simulink model "task_4"  (R2023b)
settings: Solver=FixedStepDiscrete  StartTime=0.0  StopTime=(16+14)*16-1  RelTol=1e-3
libraries: dspsigops x2, commchan3 x1, dspstat3 x1, dspsrcs4 x1
settings Model: Creator=bhalaaj  LastModifiedBy=AMEY THAKUR

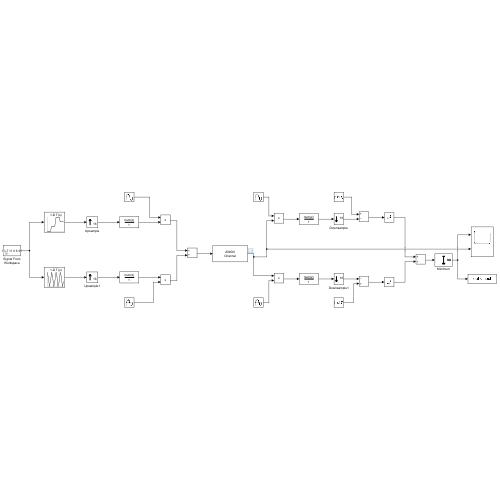
[thumbnail: Simulink's stored preview of the top-level diagram]
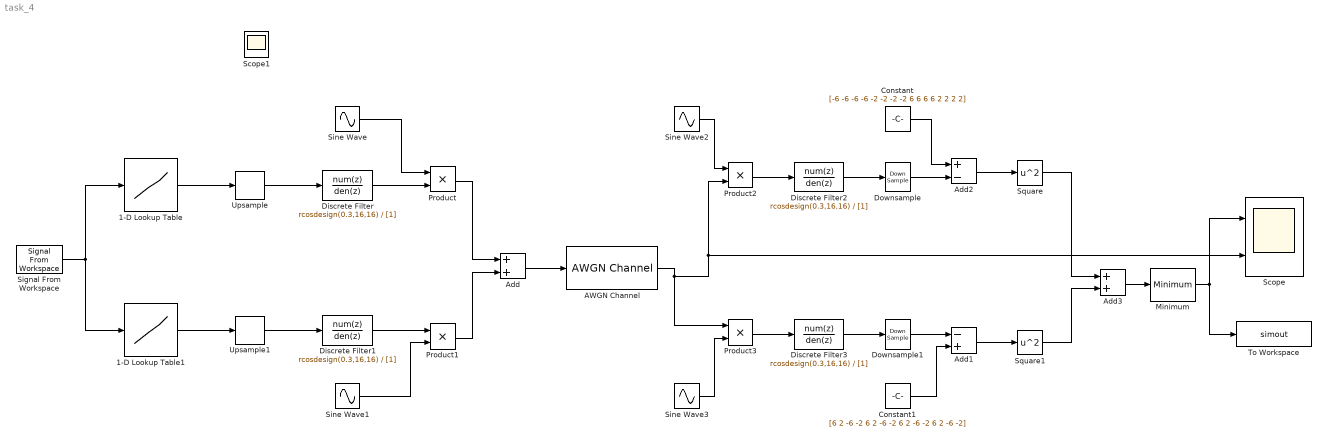
== system task_4 ==
  1-D Lookup Table : Lookup_n-D  NumberOfTableDimensions=1  BreakpointsForDimension1=[0:15]  Table=[-6 -6 -6 -6 -2 -2 -2 -2 6 6 6 6 2 2 2 2]  InternalRulePriority=Speed  RndMeth=Simplest
  1-D Lookup Table1 : Lookup_n-D  NumberOfTableDimensions=1  BreakpointsForDimension1=[0:15]  Table=[6 2 -6 -2 6 2 -6 -2 6 2 -6 -2 6 2 -6 -2]  InternalRulePriority=Speed  RndMeth=Simplest
  AWGN Channel : commchan3/AWGN Channel  LegacyMode=off  NoiseMethod="Signal to noise ratio  (Es/No)"  noiseMode="Signal to noise ratio  (SNR)"  EbNo=10  EsNo=40  SNR=10  BitsPerSymbol=1  SignalPower=1  SamplesPerSymbol=1  SymbolPeriod=1  VarianceSource=Parameter  Variance=1  RandomStream=mt19937ar with seed  Seed=110107589  SimulateUsing=Code generation
  Add : Sum
  Add1 : Sum  Inputs=-+
  Add2 : Sum  Inputs=+-
  Add3 : Sum
  Constant : Constant  Value=[-6 -6 -6 -6 -2 -2 -2 -2 6 6 6 6 2 2 2 2]
  Constant1 : Constant  Value=[6 2 -6 -2 6 2 -6 -2 6 2 -6 -2 6 2 -6 -2]
  Discrete Filter{,1..3} (4 alike) : DiscreteFilter  Numerator=rcosdesign(0.3,16,16)  Denominator=[1]
  Downsample : DownSample  N=16  RateOptions=Allow multirate processing
  Downsample1 : DownSample  N=16  RateOptions=Allow multirate processing
  Minimum : dspstat3/Minimum  operation=minimum  fcn=Index  indexBase=Zero  operateOver=Entire input  Dimension=1  InputProcessing=Columns as channels (frame based)  reset=None  roiEnable=off  roiType=Rectangles  roiPortion=Entire ROI  roiOutput=Individual statistics for each ROI  roiFlag=off  roundingMode=Floor  overflowMode=off
      settings: LibrarySourceBlock=dsphdlsupportstat/Minimum
  Product{,1..3} (4 alike) : Product
  Scope : Scope  NumInputPorts=2
  Signal From Workspace : dspsrcs4/Signal From Workspace  X=[15 13 10 3 7 11 0 6 9 3 1 2 4 5]  Ts=16  nsamps=1  OutputAfterFinalValue=Setting to zero  ignoreOrWarnInputAndFrameLengths=off  OutputFrames=off
  Sine Wave : Sin  Amplitude=sqrt(2)  Frequency=0.5*pi  Phase=pi/2  SampleTime=1
  Sine Wave1 : Sin  Amplitude=-sqrt(2)  Frequency=0.5*pi  SampleTime=1
  Sine Wave2 : Sin  Amplitude=sqrt(2)  Frequency=0.5*pi  Phase=pi/2  SampleTime=1
  Sine Wave3 : Sin  Amplitude=-sqrt(2)  Frequency=0.5*pi  SampleTime=1
  Square : Math  Operator=square
  Square1 : Math  Operator=square
  To Workspace : ToWorkspace  VariableName=simout  SampleTime=-1
      settings: Save2DSignal=2-D array (concatenate along first dimension)
  Upsample : dspsigops/Upsample  FactorSource=Dialog parameter  N=16  Nmax=16  phase=0  RateOptions=Allow multirate processing  ic=0  mode=Unused parameter value
      settings: LibrarySourceBlock=dsphdlsupportsigops/Upsample
  Upsample1 : dspsigops/Upsample  FactorSource=Dialog parameter  N=16  Nmax=16  phase=0  RateOptions=Allow multirate processing  ic=0  mode=Unused parameter value
      settings: LibrarySourceBlock=dsphdlsupportsigops/Upsample
  Scope1 : Scope
  wires:
  Signal From Workspace/1 -> 1-D Lookup Table1/1, 1-D Lookup Table/1
  1-D Lookup Table/1 -> Upsample/1
  1-D Lookup Table1/1 -> Upsample1/1
  Upsample/1 -> Discrete Filter/1
  Upsample1/1 -> Discrete Filter1/1
  Discrete Filter/1 -> Product/2
  Discrete Filter1/1 -> Product1/1
  Sine Wave/1 -> Product/1
  Sine Wave1/1 -> Product1/2
  Product/1 -> Add/1
  Product1/1 -> Add/2
  Add/1 -> AWGN Channel/1
  Sine Wave2/1 -> Product2/1
  Sine Wave3/1 -> Product3/2
  AWGN Channel/1 -> Product2/2, Scope/2, Product3/1
  Product2/1 -> Discrete Filter2/1
  Product3/1 -> Discrete Filter3/1
  Discrete Filter2/1 -> Downsample/1
  Discrete Filter3/1 -> Downsample1/1
  Downsample/1 -> Add2/2
  Downsample1/1 -> Add1/1
  Add2/1 -> Square/1
  Add1/1 -> Square1/1
  Square/1 -> Add3/1
  Square1/1 -> Add3/2
  Add3/1 -> Minimum/1
  Minimum/1 -> Scope/1, To Workspace/1
  Constant/1 -> Add2/1
  Constant1/1 -> Add1/2
